simulink model "EV_open_loop"  (Simulink 10.3)
settings: Solver=ode4  StartTime=0.0  StopTime=200  FixedStep=0.01  RelTol=1e-3
settings Model: Creator=APCL ACER 01  LastModifiedBy=APCL ACER 01
settings SolverCC: AlgebraicLoopSolver=Auto
settings DataIOCC: SaveFormat=Dataset  SignalLoggingSaveFormat=Dataset  ReturnWorkspaceOutputs=on
settings OptimizationCC: ExpressionDepthLimit=128  LifeSpan=auto
settings DebuggingCC: UnderspecifiedInitializationDetection=Simplified  MergeDetectMultiDrivingBlocksExec=error  FcnCallInpInsideContextMsg=error  UnconnectedInputMsg=none  UnconnectedOutputMsg=none  UnconnectedLineMsg=none  StateNameClashWarn=none  SFUnexpectedBacktrackingDiag=error  SFNoUnconditionalDefaultTransitionDiag=error  SFExecutionAtInitializationDiag=warning  ArithmeticOperatorsInVariantConditions=error
settings HardwareCC: ProdBitPerPointer=64  ProdBitPerSizeT=64  ProdBitPerPtrDiffT=64  ProdLargestAtomicFloat=Float  ProdIntDivRoundTo=Zero  ProdEndianess=LittleEndian  ProdWordSize=64  ProdHWDeviceType=Intel->x86-64 (Windows64)
settings ModelReferenceCC: EnableRefExpFcnMdlSchedulingChecks=off  PropagateSignalLabelsOutOfModel=on
settings SFSimCC: SimUseLocalCustomCode=on  CustomCodeUndefinedFunction=FilterOut
settings RTWCC: RTWUseLocalCustomCode=on  DLArmComputeVersion=20.02.1
settings CodeAppCC: StateflowObjectComments=off
settings GRTTargetCC: TargetLangStandard=C99 (ISO)  CombineOutputUpdateFcns=on  GRTInterface=off
settings ConfigComp: CovMetricSettings=dwe  CovSaveCumulativeToWorkspaceVar=off  CovSaveSingleToWorkspaceVar=off  CovExternalEMLEnable=on

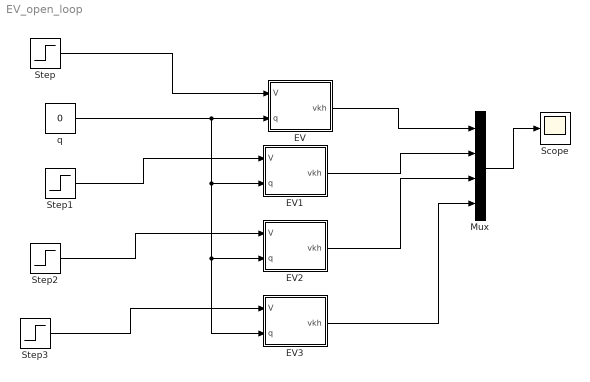
== system EV_open_loop ==
  EV : Subsystem
  EV1 : Subsystem
  EV2 : Subsystem
  EV3 : Subsystem
  Mux : Mux
  Scope : Scope
  Step : Step  Time=0  After=48  SampleTime=0
  Step1 : Step  Time=0  After=40  SampleTime=0
  Step2 : Step  Time=0  After=32  SampleTime=0
  Step3 : Step  Time=0  After=24  SampleTime=0
  q : Constant  Value=0
  wires:
  Step/1 -> EV/1(V)
  q/1 -> EV3/2(q), EV2/2(q), EV1/2(q), EV/2(q)
  Mux/1 -> Scope/1
  Step3/1 -> EV3/1(V)
  Step2/1 -> EV2/1(V)
  Step1/1 -> EV1/1(V)
  EV/1(vkh) -> Mux/1
  EV1/1(vkh) -> Mux/2
  EV2/1(vkh) -> Mux/3
  EV3/1(vkh) -> Mux/4

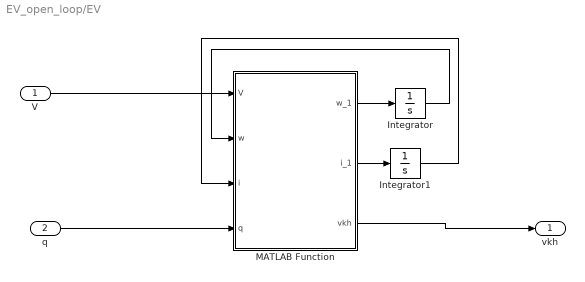
== system EV_open_loop/EV ==
  V : Inport
  q : Inport  Port=2
  Integrator : Integrator
  Integrator1 : Integrator
  MATLAB Function : MATLAB Function  TreatAsAtomicUnit=on
  vkh : Outport
  wires:
  q/1 -> MATLAB Function/4(q)
  MATLAB Function/2(i_1) -> Integrator1/1
  MATLAB Function/1(w_1) -> Integrator/1
  Integrator1/1 -> MATLAB Function/3(i)
  MATLAB Function/3(vkh) -> vkh/1
  V/1 -> MATLAB Function/1(V)
  Integrator/1 -> MATLAB Function/2(w)

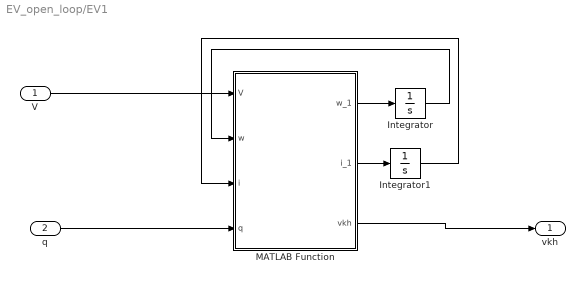
== system EV_open_loop/EV1 ==
  V : Inport
  q : Inport  Port=2
  Integrator : Integrator
  Integrator1 : Integrator
  MATLAB Function : MATLAB Function  TreatAsAtomicUnit=on
  vkh : Outport
  wires:
  Integrator/1 -> MATLAB Function/2(w)
  V/1 -> MATLAB Function/1(V)
  MATLAB Function/3(vkh) -> vkh/1
  Integrator1/1 -> MATLAB Function/3(i)
  MATLAB Function/1(w_1) -> Integrator/1
  MATLAB Function/2(i_1) -> Integrator1/1
  q/1 -> MATLAB Function/4(q)

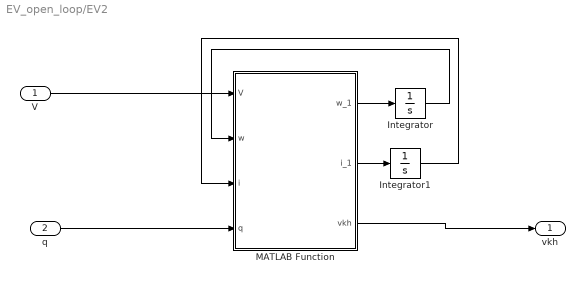
== system EV_open_loop/EV2 ==
  V : Inport
  q : Inport  Port=2
  Integrator : Integrator
  Integrator1 : Integrator
  MATLAB Function : MATLAB Function  TreatAsAtomicUnit=on
  vkh : Outport
  wires:
  q/1 -> MATLAB Function/4(q)
  MATLAB Function/2(i_1) -> Integrator1/1
  MATLAB Function/1(w_1) -> Integrator/1
  Integrator1/1 -> MATLAB Function/3(i)
  MATLAB Function/3(vkh) -> vkh/1
  V/1 -> MATLAB Function/1(V)
  Integrator/1 -> MATLAB Function/2(w)

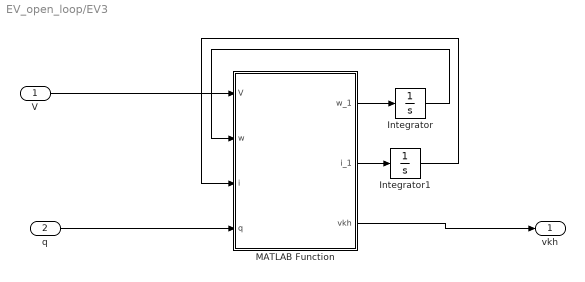
== system EV_open_loop/EV3 ==
  V : Inport
  q : Inport  Port=2
  Integrator : Integrator
  Integrator1 : Integrator
  MATLAB Function : MATLAB Function  TreatAsAtomicUnit=on
  vkh : Outport
  wires:
  Integrator/1 -> MATLAB Function/2(w)
  V/1 -> MATLAB Function/1(V)
  MATLAB Function/3(vkh) -> vkh/1
  Integrator1/1 -> MATLAB Function/3(i)
  MATLAB Function/1(w_1) -> Integrator/1
  MATLAB Function/2(i_1) -> Integrator1/1
  q/1 -> MATLAB Function/4(q)

== matlab function EV1/MATLAB Function ==
  data: V input double; w_1 output double; w input double; i input double; q input double; i_1 output double; vkh output double
function [w_1,i_1, vkh] = fcn(V, w, i,q)
L=0.006008; % inductance (La+Lf) in henry
R=0.12; % Resistance (Ra+Rf) in ohm
B=0.0002;
J=0.05;
Laf=0.001766;
m=800;
A=1.8;
rho=1.25;
Cd=0.3;
r=0.3;
N=11;
mu=0.015;
g=9.8;


v=(w*r)/N;
i_1=(1/L)*(V-R*i-Laf*i*w);

%w_1=(1/J)*(Laf*i*i-B*w-T_l);
w_1=(1/(J+m*(r/N)*(r/N)))*(Laf*i*i-B*w-(r/N)*(mu*m*g+0.5*rho*A*Cd*v*v+m*g*sin(q*pi/180)));

vkh=v*3.6;

== matlab function EV/MATLAB Function ==
  data: V input double; w_1 output double; w input double; i input double; q input double; i_1 output double; vkh output double
function [w_1,i_1, vkh] = fcn(V, w, i,q)
L=0.006008; % inductance (La+Lf) in henry
R=0.12; % Resistance (Ra+Rf) in ohm
B=0.0002;
J=0.05;
Laf=0.001766;
m=800;
A=1.8;
rho=1.25;
Cd=0.3;
r=0.3;
N=11;
mu=0.015;
g=9.8;


v=(w*r)/N;
i_1=(1/L)*(V-R*i-Laf*i*w);

%w_1=(1/J)*(Laf*i*i-B*w-T_l);
w_1=(1/(J+m*(r/N)*(r/N)))*(Laf*i*i-B*w-(r/N)*(mu*m*g+0.5*rho*A*Cd*v*v+m*g*sin(q*pi/180)));

vkh=v*3.6;

== matlab function EV2/MATLAB Function ==
  data: V input double; w_1 output double; w input double; i input double; q input double; i_1 output double; vkh output double
function [w_1,i_1, vkh] = fcn(V, w, i,q)
L=0.006008; % inductance (La+Lf) in henry
R=0.12; % Resistance (Ra+Rf) in ohm
B=0.0002;
J=0.05;
Laf=0.001766;
m=800;
A=1.8;
rho=1.25;
Cd=0.3;
r=0.3;
N=11;
mu=0.015;
g=9.8;


v=(w*r)/N;
i_1=(1/L)*(V-R*i-Laf*i*w);

%w_1=(1/J)*(Laf*i*i-B*w-T_l);
w_1=(1/(J+m*(r/N)*(r/N)))*(Laf*i*i-B*w-(r/N)*(mu*m*g+0.5*rho*A*Cd*v*v+m*g*sin(q*pi/180)));

vkh=v*3.6;

== matlab function EV3/MATLAB Function ==
  data: V input double; w_1 output double; w input double; i input double; q input double; i_1 output double; vkh output double
function [w_1,i_1, vkh] = fcn(V, w, i,q)
L=0.006008; % inductance (La+Lf) in henry
R=0.12; % Resistance (Ra+Rf) in ohm
B=0.0002;
J=0.05;
Laf=0.001766;
m=800;
A=1.8;
rho=1.25;
Cd=0.3;
r=0.3;
N=11;
mu=0.015;
g=9.8;


v=(w*r)/N;
i_1=(1/L)*(V-R*i-Laf*i*w);

%w_1=(1/J)*(Laf*i*i-B*w-T_l);
w_1=(1/(J+m*(r/N)*(r/N)))*(Laf*i*i-B*w-(r/N)*(mu*m*g+0.5*rho*A*Cd*v*v+m*g*sin(q*pi/180)));

vkh=v*3.6;
